simulink model "lecturaLaser"  (R2014a)
settings: Solver=ode45  StartTime=0.0  StopTime=Inf  RelTol=1e-3
InitFcn:
  | Ts=0.01
  | lid = LIDAR();
  | rob = DifferentialRobot();
  | rob.dt = Ts;
  | rob.attachLidar(lid, [0.6,0,0]);
  | close all;
  | figure;
  | axis equal;
  | hold on;
  | whitebg([0 0 0]);
  | grid on;
  | axis([-5 5 -5 5]);
  | view(-90, 90)
  | set(gca, 'ydir', 'reverse'); pl = Plotter(gca);
libraries: iWalkerLib x1
settings Model: Creator=Brian  LastModifiedBy=Brian

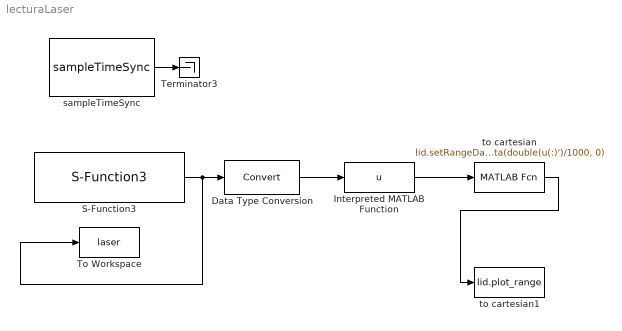
== system lecturaLaser ==
  Data Type Conversion : DataTypeConversion
  Interpreted MATLAB Function : MATLABFcn  MATLABFcn=u  SampleTime=0.5
  S-Function3 : iWalkerLib/S-Function3  mask{COM=3, SampleTime=0.2}
      mask prompts: SampleTime "Sample time"
  Terminator3 : Terminator
  To Workspace : ToWorkspace  VariableName=laser  SaveFormat=Timeseries  SampleTime=-1
  sampleTimeSync : S-Function  Priority=8  FunctionName=sampleTimeSync  EnableBusSupport=off
  to cartesian : MATLABFcn  MATLABFcn=lid.setRangeData(double(u(:)')/1000, 0)
  to cartesian1 : MATLABFcn  MATLABFcn=lid.plot_range  OutputDimensions=0  Output1D=off
  wires:
  sampleTimeSync/1 -> Terminator3/1
  Data Type Conversion/1 -> Interpreted MATLAB Function/1
  to cartesian/1 -> to cartesian1/1
  S-Function3/1 -> To Workspace/1, Data Type Conversion/1
  Interpreted MATLAB Function/1 -> to cartesian/1
